simulink model "motor_sim_signal_injection"  (R2016a)
settings: Solver=FixedStepAuto  StartTime=0.0  StopTime=.5  FixedStep=.000001  MaxStep=.00001  RelTol=1e-3
values from neighbouring files (symbols this model uses):
  F = 1e-7    (= 1e-07)    [dynamic_sim_constants.m]
  J = 1e-9    (= 1e-09)    [dynamic_sim_constants.m]
  Ki_d = 0.00001    (= 1e-05)    [dynamic_sim_constants.m]
  Ki_q = 0.00001    (= 1e-05)    [dynamic_sim_constants.m]
  Km = .00149    (= 0.00149)    [dynamic_sim_constants.m]
  Kp_d = 10    [dynamic_sim_constants.m]
  Kp_q = 10    [dynamic_sim_constants.m]
  L = 0.00001462*3/2    (= 2.193e-05)    [dynamic_sim_constants.m]    (also in serial_bin_log.m = length(log))
  P = 2    [dynamic_sim_constants.m]    (also in foc_matlab_plot.m = mean(avg_st); serial_bin_log.m = mean(avg_st); slow_1hz_current_data_2_1A.mat = 0.00101490868431; slow_1hz_current_datas.mat = 0.00101490868431)
  psi = 0.00152788745    [dynamic_sim_constants.m]
  R = .86*3/2    (= 1.29)    [dynamic_sim_constants.m]
  wc = 1000    [dynamic_sim_constants.m]
libraries: dsparch4 x2, dspfdesign x1
settings Model: Creator=Ocanath  LastModifiedBy=Ocanath

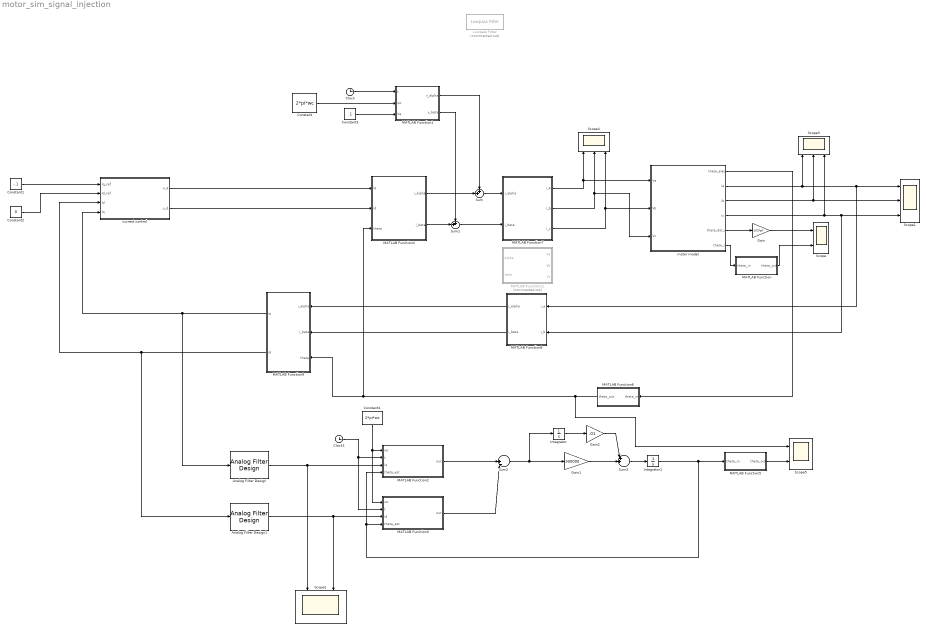
== system motor_sim_signal_injection ==
  Analog Filter Design : dsparch4/Analog Filter Design  method=Butterworth  filttype=Bandpass  N=8  Wlo=900*2*pi  Whi=1100*2*pi  Rp=2  Rs=40
  Analog Filter Design1 : dsparch4/Analog Filter Design  method=Butterworth  filttype=Bandpass  N=8  Wlo=900*2*pi  Whi=1100*2*pi  Rp=2  Rs=40
  Clock : Clock
      settings: Decimation=2000
  Clock1 : Clock
      settings: Decimation=10000
  Constant : Constant  Value=2*pi*wc
  Constant1 : Constant  Value=-.1
  Constant2 : Constant  Value=0
  Constant3 : Constant  Value=.1
  Constant4 : Constant  Value=2*pi*wc
  Gain : Gain  Gain=1/(2*pi)
  Gain1 : Gain  Gain=300000
  Gain2 : Gain  Gain=.01
  Integrator : Integrator
  Integrator1 : Integrator
  Lowpass Filter : dspfdesign/Lowpass Filter  Commented=on  FilterType=FIR  DesignForMinimumOrder=on  FilterOrder=50  PassbandFrequency=8e3  StopbandFrequency=12e3  PassbandRipple=0.1  StopbandAttenuation=80  InheritSampleRate=off  SampleRate=44100  roundingMode=Floor  coeffsDataTypeStr=fixdt(1,16)  SimulateUsing=Interpreted execution
  MATLAB Function : MATLAB Function  TreatAsAtomicUnit=on
  MATLAB Function1 : MATLAB Function  TreatAsAtomicUnit=on
  MATLAB Function11 : MATLAB Function  Commented=on  TreatAsAtomicUnit=on
  MATLAB Function2 : MATLAB Function  TreatAsAtomicUnit=on
  MATLAB Function3 : MATLAB Function  TreatAsAtomicUnit=on
  MATLAB Function4 : MATLAB Function  TreatAsAtomicUnit=on
  MATLAB Function5 : MATLAB Function  TreatAsAtomicUnit=on
  MATLAB Function6 : MATLAB Function  TreatAsAtomicUnit=on
  MATLAB Function7 : MATLAB Function  TreatAsAtomicUnit=on
  MATLAB Function8 : MATLAB Function  TreatAsAtomicUnit=on
  MATLAB Function9 : MATLAB Function  TreatAsAtomicUnit=on
  Scope : Scope  NumInputPorts=2
  Scope1 : Scope  NumInputPorts=3
  Scope2 : Scope  NumInputPorts=2
  Scope3 : Scope  NumInputPorts=3
  Scope4 : Scope  NumInputPorts=3
  Scope5 : Scope  NumInputPorts=2
  Sum : Sum  Inputs=++|
  Sum1 : Sum  Inputs=++|
  Sum2 : Sum  Inputs=||+-|
  Sum3 : Sum  Inputs=|++||
  "current control " : Subsystem
  "motor model " : Subsystem
  wires:
  MATLAB Function7/1(i_a) -> Scope4/1, "motor model "/1("Va ")
  "motor model "/5(theta_dot_r) -> Gain/1
  MATLAB Function8/2(i_beta) -> MATLAB Function9/2(i_beta)
  MATLAB Function8/1(i_alpha) -> MATLAB Function9/1(i_alpha)
  "motor model "/6(theta_r) -> MATLAB Function/1(theta_in)
  MATLAB Function/1(theta_out) -> Scope/2
  Gain/1 -> Scope/1
  MATLAB Function7/2(i_b) -> "motor model "/3(Vc), Scope4/2
  MATLAB Function7/3(i_c) -> Scope4/3, "motor model "/2(Vb)
  "motor model "/3(ib) -> Scope3/2, Scope1/2
  "motor model "/1(" theta_elec ") -> MATLAB Function6/1(theta_in)
  "motor model "/4(ic) -> Scope3/3, Scope1/3, MATLAB Function8/2(i_b)
  "motor model "/2(ia) -> Scope3/1, MATLAB Function8/1(i_a), Scope1/1
  Constant1/1 -> "current control "/1(Iq_ref)
  Constant2/1 -> "current control "/2(Id_ref)
  "current control "/1(u_q) -> MATLAB Function4/1(iq)
  Constant/1 -> MATLAB Function1/2(wc)
  "current control "/2(u_d) -> MATLAB Function4/2(id)
  Sum1/1 -> MATLAB Function7/2(i_beta)
  Sum/1 -> MATLAB Function7/1(i_alpha)
  MATLAB Function4/1(i_alpha) -> Sum/2
  MATLAB Function4/2(i_beta) -> Sum1/2
  Constant3/1 -> MATLAB Function1/3(Va)
  Clock/1 -> MATLAB Function1/1(t)
  MATLAB Function1/2(v_beta) -> Sum1/1
  MATLAB Function1/1(v_alpha) -> Sum/1
  MATLAB Function9/1(iq) -> Analog Filter Design/1, "current control "/4(Iq)
  MATLAB Function9/2(id) -> Analog Filter Design1/1, "current control "/3(Id)
  Analog Filter Design/1 -> MATLAB Function2/3(iq), Scope2/1
  Analog Filter Design1/1 -> MATLAB Function3/3(id), Scope2/2
  Gain1/1 -> Sum3/2
  Clock1/1 -> MATLAB Function2/2(t), MATLAB Function3/2(t)
  Constant4/1 -> MATLAB Function2/1(wc), MATLAB Function3/1(wc)
  MATLAB Function2/1(out) -> Sum2/1
  MATLAB Function3/1(out) -> Sum2/2
  Sum2/1 -> Integrator/1, Gain1/1
  Integrator/1 -> Gain2/1
  Gain2/1 -> Sum3/1
  Sum3/1 -> Integrator1/1
  Integrator1/1 -> MATLAB Function3/4(theta_est), MATLAB Function2/4(theta_est), MATLAB Function5/1(theta_in)
  MATLAB Function5/1(theta_out) -> Scope5/2
  MATLAB Function6/1(theta_out) -> Scope5/1, MATLAB Function9/3(theta), MATLAB Function4/3(theta)

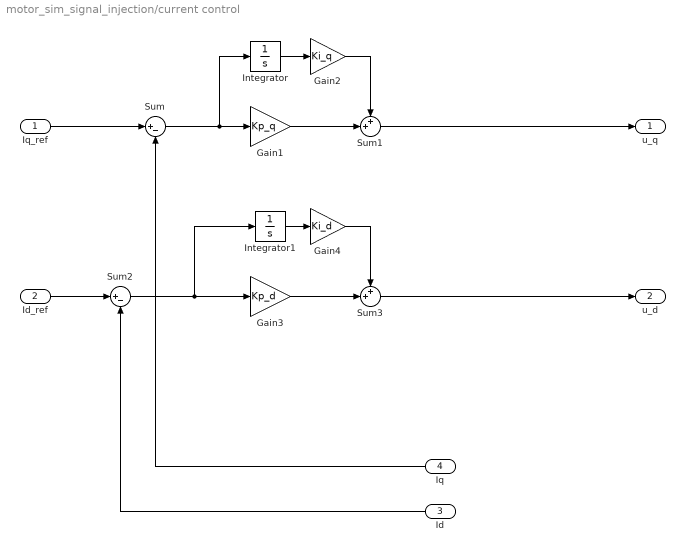
== system motor_sim_signal_injection/current control  ==
  Iq_ref : Inport
  Id_ref : Inport  Port=2
  Id : Inport  Port=3
  Iq : Inport  Port=4
  Gain1 : Gain  Gain=Kp_q
  Gain2 : Gain  Gain=Ki_q
  Gain3 : Gain  Gain=Kp_d
  Gain4 : Gain  Gain=Ki_d
  Integrator : Integrator
  Integrator1 : Integrator
  Sum : Sum  Inputs=|+-
  Sum1 : Sum  Inputs=++|
  Sum2 : Sum  Inputs=|+-
  Sum3 : Sum  Inputs=++|
  u_q : Outport
  u_d : Outport  Port=2
  wires:
  Id_ref/1 -> Sum2/1
  Sum/1 -> Integrator/1, Gain1/1
  Integrator/1 -> Gain2/1
  Gain1/1 -> Sum1/2
  Iq_ref/1 -> Sum/1
  Gain2/1 -> Sum1/1
  Sum1/1 -> u_q/1
  Gain4/1 -> Sum3/1
  Sum2/1 -> Integrator1/1, Gain3/1
  Integrator1/1 -> Gain4/1
  Id/1 -> Sum2/2
  Iq/1 -> Sum/2
  Sum3/1 -> u_d/1
  Gain3/1 -> Sum3/2

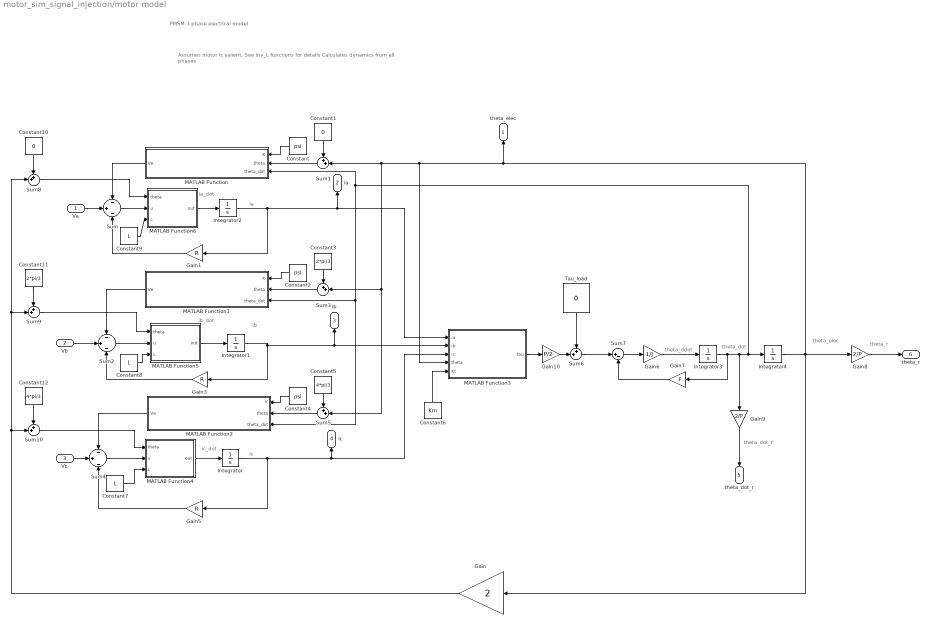
== system motor_sim_signal_injection/motor model  ==
  note: Assumes motor is salient. See inv_L functions for details
      | Calculates dynamics from all phases
  note: PMSM 3 phase electrical model
  note: theta_dot_r
  note: theta_r
  note: theta_elec
  note: theta_dot
  note: theta_ddot
  note: ia
  note: ia_dot
  note: ib
  note: ib_dot
  note: ic
  note: ic_dot
  "Va " : Inport
  Vb : Inport  Port=2
  Vc : Inport  Port=3
  Constant : Constant  Value=psi
  Constant1 : Constant  Value=0
  Constant10 : Constant  Value=0
  Constant11 : Constant  Value=2*pi/3
  Constant12 : Constant  Value=4*pi/3
  Constant2 : Constant  Value=psi
  Constant3 : Constant  Value=2*pi/3
  Constant4 : Constant  Value=psi
  Constant5 : Constant  Value=4*pi/3
  Constant6 : Constant  Value=Km
  Constant7 : Constant  Value=L
  Constant8 : Constant  Value=L
  Constant9 : Constant  Value=L
  Gain : Gain  Gain=2
  Gain1 : Gain  Gain=R
  Gain10 : Gain  Gain=P/2
  Gain3 : Gain  Gain=R
  Gain5 : Gain  Gain=R
  Gain6 : Gain  Gain=1/J
  Gain7 : Gain  Gain=F
  Gain8 : Gain  Gain=2/P
  Gain9 : Gain  Gain=2/P
  Integrator{,1..4} (5 alike) : Integrator
  MATLAB Function : MATLAB Function  TreatAsAtomicUnit=on
  MATLAB Function1 : MATLAB Function  TreatAsAtomicUnit=on
  MATLAB Function2 : MATLAB Function  TreatAsAtomicUnit=on
  MATLAB Function3 : MATLAB Function  TreatAsAtomicUnit=on
  MATLAB Function4 : MATLAB Function  TreatAsAtomicUnit=on
  MATLAB Function5 : MATLAB Function  TreatAsAtomicUnit=on
  MATLAB Function6 : MATLAB Function  TreatAsAtomicUnit=on
  Sum : Sum  Inputs=-|+|-
  Sum{1,3,5..6,8..10} (7 alike) : Sum  Inputs=++|
  Sum2 : Sum  Inputs=-|+|-
  Sum4 : Sum  Inputs=-|+|-
  Sum7 : Sum  Inputs=|+-
  Tau_load : Constant  Value=0
  " theta_elec " : Outport
  ia : Outport  Port=2
  ib : Outport  Port=3
  ic : Outport  Port=4
  theta_dot_r : Outport  Port=5
  theta_r : Outport  Port=6
  wires:
  Sum6/1 -> Sum7/1
  Gain5/1 -> Sum4/3
  Integrator2/1 -> Gain1/1, ia/1, MATLAB Function3/1(ia)
  Constant6/1 -> MATLAB Function3/5(Kt)
  Integrator/1 -> Gain5/1, ic/1, MATLAB Function3/3(ic)
  MATLAB Function1/1(Ve) -> Sum2/1
  MATLAB Function2/1(Ve) -> Sum4/1
  Gain3/1 -> Sum2/3
  Integrator1/1 -> Gain3/1, ib/1, MATLAB Function3/2(ib)
  Constant/1 -> MATLAB Function/1(K)
  Constant2/1 -> MATLAB Function1/1(K)
  Constant3/1 -> Sum3/1
  Gain1/1 -> Sum/3
  Constant4/1 -> MATLAB Function2/1(K)
  Integrator3/1 -> Integrator4/1, MATLAB Function2/3(theta_dot), MATLAB Function1/3(theta_dot), MATLAB Function/3(theta_dot), Gain9/1, Gain7/1
  Constant1/1 -> Sum1/1
  Constant5/1 -> Sum5/1
  MATLAB Function3/1(tau) -> Gain10/1
  MATLAB Function/1(Ve) -> Sum/1
  Tau_load/1 -> Sum6/1
  Gain8/1 -> theta_r/1
  Sum7/1 -> Gain6/1
  Gain6/1 -> Integrator3/1
  Gain9/1 -> theta_dot_r/1
  Vc/1 -> Sum4/2
  Vb/1 -> Sum2/2
  "Va "/1 -> Sum/2
  Gain7/1 -> Sum7/2
  Gain10/1 -> Sum6/2
  Sum4/1 -> MATLAB Function4/2(u)
  MATLAB Function4/1(out) -> Integrator/1
  Constant7/1 -> MATLAB Function4/3(L)
  Sum5/1 -> MATLAB Function2/2(theta)
  Sum2/1 -> MATLAB Function5/2(u)
  MATLAB Function5/1(out) -> Integrator1/1
  Constant8/1 -> MATLAB Function5/3(L)
  Sum3/1 -> MATLAB Function1/2(theta)
  Sum/1 -> MATLAB Function6/2(u)
  MATLAB Function6/1(out) -> Integrator2/1
  Sum1/1 -> MATLAB Function/2(theta)
  Constant9/1 -> MATLAB Function6/3(L)
  Integrator4/1 -> Gain/1, Gain8/1, Sum1/2, Sum5/2, Sum3/2, MATLAB Function3/4(theta), " theta_elec "/1
  Sum8/1 -> MATLAB Function6/1(theta)
  Constant10/1 -> Sum8/1
  Sum9/1 -> MATLAB Function5/1(theta)
  Sum10/1 -> MATLAB Function4/1(theta)
  Constant11/1 -> Sum9/1
  Constant12/1 -> Sum10/1
  Gain/1 -> Sum8/2, Sum9/2, Sum10/2

== matlab function motor_sim_signal_injection/motor model /MATLAB Function1 ==
  data: K input; Ve output; theta input; theta_dot input
function Ve = emf(K,theta,theta_dot)
%#codegen
Ve = K*sin(theta)*theta_dot;
end

== matlab function motor_sim_signal_injection/motor model /MATLAB Function ==
  data: K input; Ve output; theta input; theta_dot input
function Ve = emf(K,theta,theta_dot)
%#codegen
Ve = K*sin(theta)*theta_dot;
end

== matlab function motor_sim_signal_injection/motor model /MATLAB Function2 ==
  data: K input; theta input; theta_dot input; Ve output
function Ve = emf(K,theta,theta_dot)
%#codegen
Ve = K*sin(theta)*theta_dot;
end

== matlab function motor_sim_signal_injection/motor model /MATLAB Function3 ==
  data: ia input; tau output; ib input; ic input; theta input; Kt input
function tau = tau_elec(ia,ib,ic,theta,Kt)

tau = Kt*(ia*sin(theta) + ib*sin(theta+2*pi/3) + ic*sin(theta+4*pi/3));

end

== matlab function motor_sim_signal_injection/MATLAB Function4 ==
  data: iq input; i_alpha output; id input; theta input; i_beta output
function [i_alpha,i_beta] = inverse_park(iq, id, theta)
    sin_theta = sin(theta);
    cos_theta = cos(theta);
    i_alpha = id*cos_theta - iq*sin_theta;
	i_beta = id*sin_theta + iq*cos_theta;
end

== matlab function motor_sim_signal_injection/MATLAB Function ==
  data: theta_in input; theta_out output
function theta_out = encoder(theta_in)
theta_out = atan2(sin(theta_in),cos(theta_in));
end

== matlab function motor_sim_signal_injection/motor model /MATLAB Function5 ==
  data: theta input; out output; u input; L input
function out =  inv_L(theta, u, L)
    delta_L = L/100;
%     delta_L = 0;
    Lsal = L + delta_L*cos(theta);
    out = (1/Lsal)*u;
%     out = (1/L)*u;
end

== matlab function motor_sim_signal_injection/MATLAB Function7 ==
  data: i_alpha input; i_a output; i_beta input; i_b output; i_c output
function [i_a,i_b,i_c] = inverse_clarke(i_alpha,i_beta)
    sqrt_3_by_2 = sqrt(3)*.5;
	i_a = i_alpha;
	i_b = -.5*i_alpha + sqrt_3_by_2*i_beta;
	i_c = -.5*i_alpha - sqrt_3_by_2*i_beta;
end

== matlab function motor_sim_signal_injection/MATLAB Function8 ==
  data: i_a input; i_alpha output; i_b input; i_beta output
function [i_alpha, i_beta] = clarke(i_a, i_b)
    i_alpha = i_a;
	i_beta = (1/sqrt(3))*i_a + (2/sqrt(3))*i_b;
end

== matlab function motor_sim_signal_injection/MATLAB Function9 ==
  data: i_alpha input; iq output; i_beta input; theta input; id output
function [iq,id] = park(i_alpha, i_beta, theta)
    cos_theta = cos(theta);
    sin_theta = sin(theta);
	id = i_alpha*cos_theta+i_beta*sin_theta;
	iq = -i_alpha*sin_theta+i_beta*cos_theta;
end

== matlab function motor_sim_signal_injection/motor model /MATLAB Function6 ==
  data: theta input; out output; u input; L input
function out =  inv_L(theta, u, L)
    delta_L = L/100;
%     delta_L = 0;
    Lsal = L + delta_L*cos(theta);
    out = (1/Lsal)*u;
%     out = (1/L)*u;
end

== matlab function motor_sim_signal_injection/MATLAB Function1 ==
  data: t input; v_alpha output; wc input; v_beta output; Va input
function [v_alpha,v_beta] = injector(t, wc, Va)
v_alpha = Va*cos(wc*t);
v_beta = Va*sin(wc*t);
end

== matlab function motor_sim_signal_injection/MATLAB Function2 ==
  data: wc input; t input; iq input; theta_est input; out output
function out = heterodyne_cos(wc, t, iq, theta_est)

out = iq*cos(2*theta_est - wc*t);

end

== matlab function motor_sim_signal_injection/MATLAB Function6 ==
  data: theta_in input; theta_out output
function theta_out = encoder(theta_in)
theta_out = atan2(sin(theta_in),cos(theta_in));
end

== matlab function motor_sim_signal_injection/motor model /MATLAB Function4 ==
  data: theta input; out output; u input; L input
function out =  inv_L(theta, u, L)
    delta_L = L/100;
%     delta_L = 0;
    Lsal = L + delta_L*cos(theta);
    out = (1/Lsal)*u;
%     out = (1/L)*u;
end

== matlab function motor_sim_signal_injection/MATLAB Function11 ==
  data: alpha input; Va output; beta input; Vb output; Vc output
function [Va,Vb,Vc] = svm(alpha,beta)

	pwm_half_period = 1000;
    SQRT_3 = sqrt(3);
	if(beta >= 0.0)

		if(alpha >= 0.0)

			if(beta <= alpha*SQRT_3)
				sector = 1;
			else					
				sector = 2;  
            end
		else			
			if(beta <= alpha*-SQRT_3)	
				sector = 3;
			else							
				sector = 2;
            end
        end
	else		
		if(alpha >= 0.0)	
			if(beta < -SQRT_3*alpha)
				sector = 5;
			else
				sector = 6;
            end
		else			
			if(beta < alpha*SQRT_3)
				sector = 5;
			else
				sector = 4;
            end
        end
    end
    ONE_BY_SQRT_3 = 1/SQRT_3;
    TWO_BY_SQRT_3 = 2*ONE_BY_SQRT_3;
	switch (sector)
        case 1
            t1 = ((alpha - ONE_BY_SQRT_3 * beta) * pwm_half_period);
            t2 = ((TWO_BY_SQRT_3 * beta) * pwm_half_period);
            Va = (pwm_half_period - t1 - t2) / 2;
            Vb = Va + t1;
            Vc = Vb + t2;
        case 2
            t2 = ((alpha + ONE_BY_SQRT_3 * beta) * pwm_half_period);
            t3 = ((-alpha + ONE_BY_SQRT_3 * beta) * pwm_half_period);
            Vb = (pwm_half_period - t2 - t3) / 2;
            Va = Vb + t3;
            Vc = Va + t2;
        case 3
            t3 = ((TWO_BY_SQRT_3 * beta) * pwm_half_period);
            t4 = ((-alpha - ONE_BY_SQRT_3 * beta) * pwm_half_period);
            Vb = (pwm_half_period - t3 - t4) / 2;
            Vc = Vb + t3;
            Va = Vc + t4;
        case 4
            t4 = ((-alpha + ONE_BY_SQRT_3 * beta) * pwm_half_period);
            t5 = ((-TWO_BY_SQRT_3 * beta) * pwm_half_period);
            Vc = (pwm_half_period - t4 - t5) / 2;
            Vb = Vc + t5;
            Va = Vb + t4;
        case 5
        
            t5 = ((-alpha - ONE_BY_SQRT_3 * beta) * pwm_half_period);
            t6 = ((alpha - ONE_BY_SQRT_3 * beta) * pwm_half_period);
            Vc = (pwm_half_period - t5 - t6) / 2;
            Va = Vc + t5;
            Vb = Va + t6;
        case 6
            t6 = ((-TWO_BY_SQRT_3 * beta) * pwm_half_period);
            t1 = ((alpha + ONE_BY_SQRT_3 * beta) * pwm_half_period);
            Va = (pwm_half_period - t6 - t1) / 2;
            Vc = Va + t1;
            Vb = Vc + t6;
        otherwise
            Va = 0;
            Vb = 0;
            Vc = 0;
    end
    Va = (Va-500)*8/1000;
    Vb = (Vb-500)*8/1000;
    Vc = (Vc-500)*8/1000;
end

== matlab function motor_sim_signal_injection/MATLAB Function3 ==
  data: wc input; t input; id input; theta_est input; out output
function out = heterodyne_sin(wc, t,id,theta_est )

out = id*sin(2*theta_est - wc*t);

end

== matlab function motor_sim_signal_injection/MATLAB Function5 ==
  data: theta_in input; theta_out output
function theta_out = encoder(theta_in)
theta_out = atan2(sin(theta_in),cos(theta_in));
end
